simulink model "EnergyDemandBackward"  (R2022b)
settings: Solver=ode4  StartTime=0.0  StopTime=tCycle_s(end)  FixedStep=1  RelTol=1e-3  EnableMultiTasking=on
undefined symbols (not defined in the file or in its folder): areaVeh, distRange_km, etaRec, facCw, facRoll, g, massVeh, rhoAir, tCycle_s, velCycle_kph
libraries: simulink x2
settings Model: Creator=raschul  LastModifiedBy=schuler
settings SolverCC: AlgebraicLoopSolver=TrustRegion
settings DataIOCC: LimitDataPoints=on  SaveFormat=Array  SignalLoggingSaveFormat=ModelDataLogs  ReturnWorkspaceOutputs=off
settings OptimizationCC: ExpressionDepthLimit=2147483647  LifeSpan=inf
settings DebuggingCC: UnderspecifiedInitializationDetection=Classic  MergeDetectMultiDrivingBlocksExec=none  SolverPrmCheckMsg=warning  FcnCallInpInsideContextMsg=warning  UnconnectedInputMsg=warning  UnconnectedOutputMsg=warning  UnconnectedLineMsg=warning  AllowSymbolicDim=off  StateNameClashWarn=warning  SFUnexpectedBacktrackingDiag=warning  SFNoUnconditionalDefaultTransitionDiag=warning  SFExecutionAtInitializationDiag=none  SFMachineParentedDataDiag=warning  ArithmeticOperatorsInVariantConditions=warning
settings HardwareCC: ProdBitPerPointer=32  ProdBitPerSizeT=32  ProdBitPerPtrDiffT=32  ProdLargestAtomicFloat=None  ProdIntDivRoundTo=Undefined  ProdEndianess=Unspecified  ProdWordSize=32  ProdHWDeviceType=32-bit Generic
settings ModelReferenceCC: EnableRefExpFcnMdlSchedulingChecks=on  PropagateSignalLabelsOutOfModel=off
settings SFSimCC: SimUseLocalCustomCode=off  CustomCodeUndefinedFunction=UseInterfaceOnly
settings RTWCC: RTWUseLocalCustomCode=off
settings CodeAppCC: StateflowObjectComments=on
settings GRTTargetCC: TargetLangStandard=C89/C90 (ANSI)  CombineOutputUpdateFcns=off  GRTInterface=on
settings ConfigComp: CovMetricSettings=dw  CovSaveCumulativeToWorkspaceVar=on  CovSaveSingleToWorkspaceVar=on  CovExternalEMLEnable=off

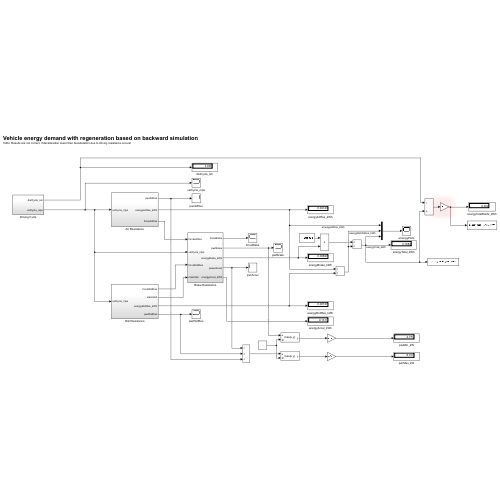
[thumbnail: Simulink's stored preview of the top-level diagram]
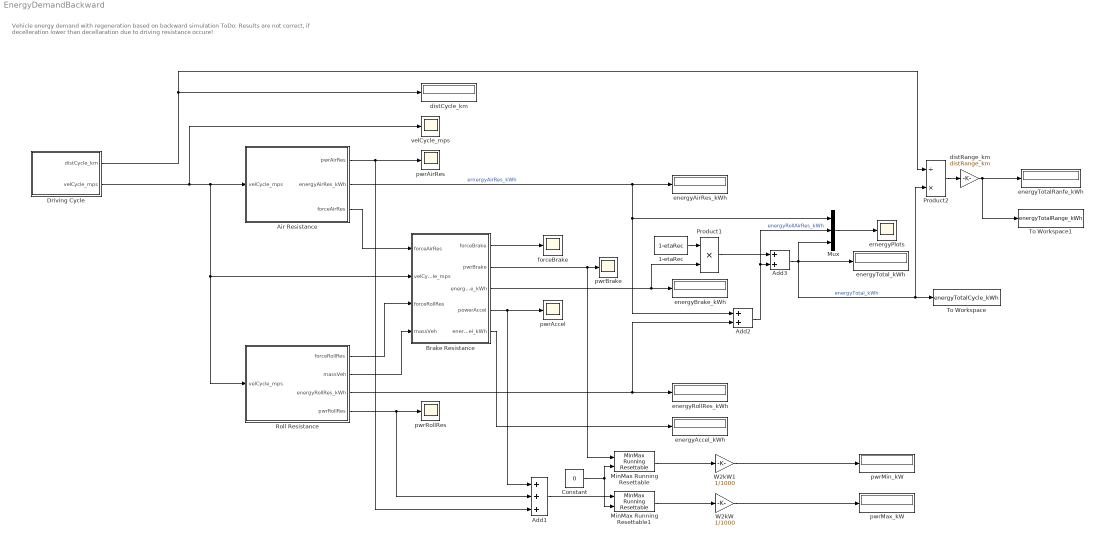
== system EnergyDemandBackward ==
  note: Vehicle energy demand with regeneration based on backward simulation
      | ToDo: Results are not correct, if decelleration lower than decellaration due to driving resistance occure!
  1-etaRec : Constant  Value=1-etaRec
  Add1 : Sum  Inputs=+++
  Add2 : Sum
  Add3 : Sum
  Air Resistance : Subsystem
  Brake Resistance : Subsystem
  Constant : Constant  Value=0
  Driving Cycle : Subsystem
  MinMax Running Resettable : simulink/Math Operations/MinMax Running Resettable  Function=max  vinit=0.0
  MinMax Running Resettable1 : simulink/Math Operations/MinMax Running Resettable  Function=max  vinit=0.0
  Mux : Mux  Inputs=3
  Product1 : Product  RndMeth=Zero
  Product2 : Product  Inputs=/*  RndMeth=Zero
  Roll Resistance : Subsystem
  To Workspace : ToWorkspace  VariableName=energyTotalCycle_kWh  SaveFormat=Timeseries  SampleTime=-1
  To Workspace1 : ToWorkspace  VariableName=energyTotalRange_kWh  SaveFormat=Timeseries  SampleTime=-1
  W2kW : Gain  Gain=1/1000
  W2kW1 : Gain  Gain=1/1000
  distCycle_km : Display
  distRange_km : Gain  Gain=distRange_km
  energyAccel_kWh : Display
  energyAirRes_kWh : Display
  energyBrake_kWh : Display
  energyRollRes_kWh : Display
  energyTotalRanfe_kWh : Display
  energyTotal_kWh : Display
  ernergyPlots : Scope
  forceBrake : Scope
  pwrAccel : Scope
  pwrAirRes : Scope
  pwrBrake : Scope
  pwrMax_kW : Display
  pwrMin_kW : Display
  pwrRollRes : Scope
  velCycle_mps : Scope
  wires:
  Driving Cycle/2(velCycle_mps) -> velCycle_mps/1, Roll Resistance/1(velCycle_mps), Brake Resistance/2(velCycle_mps), Air Resistance/1(velCycle_mps)
  Air Resistance/2(energyAirRes_kWh) -> Mux/1, Add2/1, energyAirRes_kWh/1  "ernergyAirRes_kWh"
  Roll Resistance/3(energyRollRes_kWh) -> Add2/2, energyRollRes_kWh/1
  Add2/1 -> Mux/2, Add3/2  "energyRollAirRes_kWh"
  Add3/1 -> Product2/2, To Workspace/1, Mux/3, energyTotal_kWh/1  "energyTotal_kWh"
  Mux/1 -> ernergyPlots/1
  Air Resistance/1(pwrAirRes) -> Add1/3, pwrAirRes/1
  Air Resistance/3(forceAirRes) -> Brake Resistance/1(forceAirRes)
  Roll Resistance/4(pwrRollRes) -> Add1/2, pwrRollRes/1
  Roll Resistance/1(forceRollRes) -> Brake Resistance/3(forceRollRes)
  Roll Resistance/2(massVeh) -> Brake Resistance/4(massVeh)
  Brake Resistance/1(forceBrake) -> forceBrake/1
  Brake Resistance/2(pwrBrake) -> MinMax Running Resettable/1, pwrBrake/1
  Driving Cycle/1(distCycle_km) -> Product2/1, distCycle_km/1
  Brake Resistance/4(powerAccel) -> pwrAccel/1, Add1/1
  Add1/1 -> MinMax Running Resettable1/1
  MinMax Running Resettable1/1 -> W2kW/1
  W2kW/1 -> pwrMax_kW/1
  MinMax Running Resettable/1 -> W2kW1/1
  W2kW1/1 -> pwrMin_kW/1
  Constant/1 -> MinMax Running Resettable1/2, MinMax Running Resettable/2
  Product1/1 -> Add3/1
  Brake Resistance/5(energyAccel_kWh) -> energyAccel_kWh/1
  1-etaRec/1 -> Product1/1
  Brake Resistance/3(energyBrake_kWh) -> Product1/2, energyBrake_kWh/1
  Product2/1 -> distRange_km/1
  distRange_km/1 -> To Workspace1/1, energyTotalRanfe_kWh/1

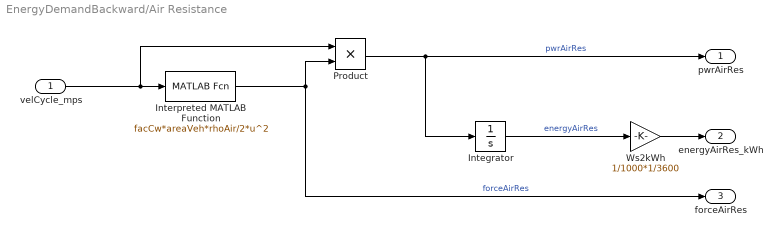
== system EnergyDemandBackward/Air Resistance ==
  velCycle_mps : Inport
  Integrator : Integrator
  Interpreted MATLAB Function : MATLABFcn  MATLABFcn=facCw*areaVeh*rhoAir/2*u^2
  Product : Product  RndMeth=Zero
  Ws2kWh : Gain  Gain=1/1000*1/3600
  pwrAirRes : Outport  VectorParamsAs1DForOutWhenUnconnected=off
  energyAirRes_kWh : Outport  Port=2  VectorParamsAs1DForOutWhenUnconnected=off
  forceAirRes : Outport  Port=3  VectorParamsAs1DForOutWhenUnconnected=off
  wires:
  Interpreted MATLAB Function/1 -> Product/2, forceAirRes/1  "forceAirRes"
  Product/1 -> Integrator/1, pwrAirRes/1  "pwrAirRes"
  Integrator/1 -> Ws2kWh/1  "energyAirRes"
  velCycle_mps/1 -> Product/1, Interpreted MATLAB Function/1
  Ws2kWh/1 -> energyAirRes_kWh/1

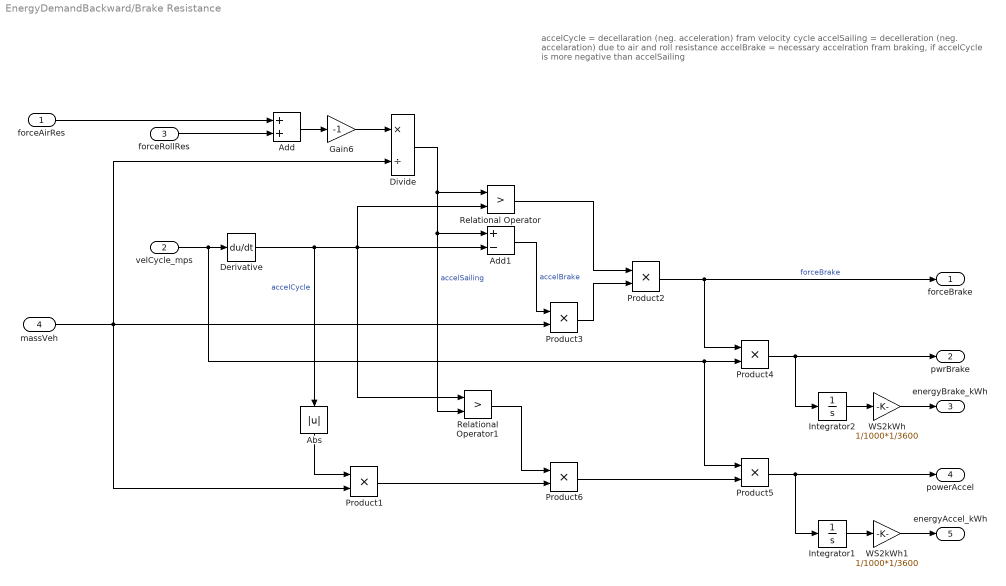
== system EnergyDemandBackward/Brake Resistance ==
  note: accelCycle = decellaration (neg. acceleration) fram velocity cycle
      | accelSailing = decelleration (neg. accelaration) due to air and roll resistance
      | accelBrake = necessary accelration fram braking, if accelCycle is more negative than accelSailing
  forceAirRes : Inport
  velCycle_mps : Inport  Port=2
  forceRollRes : Inport  Port=3
  massVeh : Inport  Port=4
  Abs : Abs  SaturateOnIntegerOverflow=off
  Add : Sum
  Add1 : Sum  Inputs=+-
  Derivative : Derivative
  Divide : Product  Inputs=*/
  Gain6 : Gain  Gain=-1
  Integrator1 : Integrator
  Integrator2 : Integrator
  Product{1..6} (6 alike) : Product  RndMeth=Zero
  Relational Operator : RelationalOperator  Operator=>  OutDataTypeStr=boolean  InputSameDT=off
  Relational Operator1 : RelationalOperator  Operator=>  OutDataTypeStr=boolean  InputSameDT=off
  WS2kWh : Gain  Gain=1/1000*1/3600
  WS2kWh1 : Gain  Gain=1/1000*1/3600
  forceBrake : Outport  VectorParamsAs1DForOutWhenUnconnected=off
  pwrBrake : Outport  Port=2  VectorParamsAs1DForOutWhenUnconnected=off
  energyBrake_kWh : Outport  Port=3  VectorParamsAs1DForOutWhenUnconnected=off
  powerAccel : Outport  Port=4  VectorParamsAs1DForOutWhenUnconnected=off
  energyAccel_kWh : Outport  Port=5  VectorParamsAs1DForOutWhenUnconnected=off
  wires:
  Derivative/1 -> Abs/1, Relational Operator1/1, Relational Operator/2, Add1/2  "accelCycle"
  Add/1 -> Gain6/1
  Gain6/1 -> Divide/1
  Divide/1 -> Relational Operator1/2, Add1/1, Relational Operator/1  "accelSailing"
  Relational Operator/1 -> Product2/1
  Add1/1 -> Product3/1  "accelBrake"
  Product3/1 -> Product2/2
  massVeh/1 -> Product1/2, Product3/2, Divide/2
  velCycle_mps/1 -> Product5/1, Product4/2, Derivative/1
  forceAirRes/1 -> Add/1
  forceRollRes/1 -> Add/2
  Product2/1 -> Product4/1, forceBrake/1  "forceBrake"
  Integrator2/1 -> WS2kWh/1
  Product4/1 -> pwrBrake/1, Integrator2/1
  WS2kWh/1 -> energyBrake_kWh/1
  Relational Operator1/1 -> Product6/1
  Product1/1 -> Product6/2
  Product6/1 -> Product5/2
  Integrator1/1 -> WS2kWh1/1
  Product5/1 -> Integrator1/1, powerAccel/1
  WS2kWh1/1 -> energyAccel_kWh/1
  Abs/1 -> Product1/1

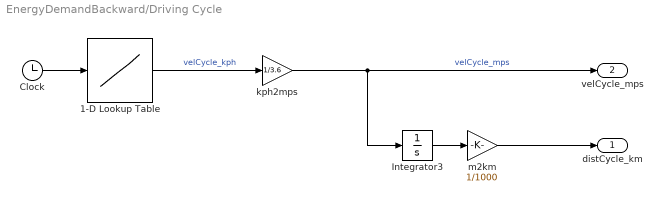
== system EnergyDemandBackward/Driving Cycle ==
  1-D Lookup Table : Lookup_n-D  NumberOfTableDimensions=1  BreakpointsForDimension1=tCycle_s  Table=velCycle_kph  RndMeth=Simplest
  Clock : Clock
  Integrator3 : Integrator
  kph2mps : Gain  Gain=1/3.6
  m2km : Gain  Gain=1/1000
  distCycle_km : Outport  VectorParamsAs1DForOutWhenUnconnected=off
  velCycle_mps : Outport  Port=2  VectorParamsAs1DForOutWhenUnconnected=off
  wires:
  1-D Lookup Table/1 -> kph2mps/1  "velCycle_kph"
  Clock/1 -> 1-D Lookup Table/1
  kph2mps/1 -> Integrator3/1, velCycle_mps/1  "velCycle_mps"
  Integrator3/1 -> m2km/1
  m2km/1 -> distCycle_km/1

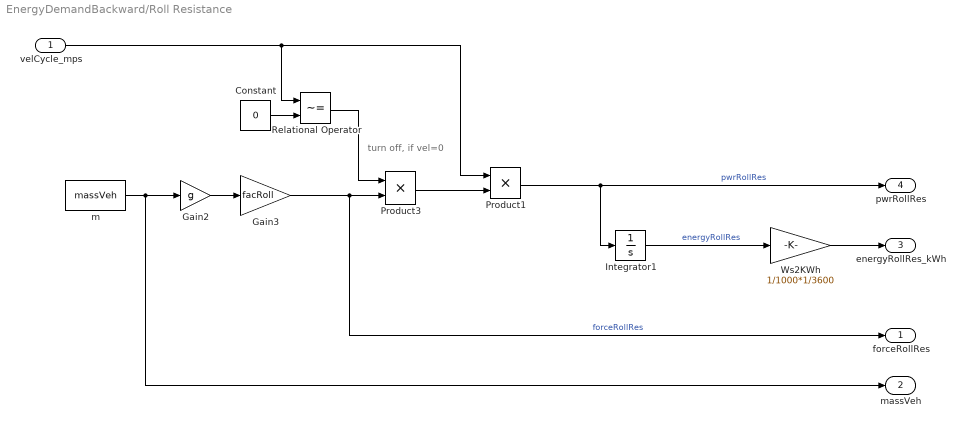
== system EnergyDemandBackward/Roll Resistance ==
  note: turn off, if vel=0
  velCycle_mps : Inport
  Constant : Constant  Value=0
  Gain2 : Gain  Gain=g
  Gain3 : Gain  Gain=facRoll
  Integrator1 : Integrator
  Product1 : Product  RndMeth=Zero
  Product3 : Product  RndMeth=Zero
  Relational Operator : RelationalOperator  Operator=~=  OutDataTypeStr=boolean  InputSameDT=off
  Ws2KWh : Gain  Gain=1/1000*1/3600
  m : Constant  Value=massVeh
  forceRollRes : Outport  VectorParamsAs1DForOutWhenUnconnected=off
  massVeh : Outport  Port=2  VectorParamsAs1DForOutWhenUnconnected=off
  energyRollRes_kWh : Outport  Port=3  VectorParamsAs1DForOutWhenUnconnected=off
  pwrRollRes : Outport  Port=4  VectorParamsAs1DForOutWhenUnconnected=off
  wires:
  m/1 -> Gain2/1, massVeh/1
  Gain2/1 -> Gain3/1
  Product1/1 -> Integrator1/1, pwrRollRes/1  "pwrRollRes"
  Integrator1/1 -> Ws2KWh/1  "energyRollRes"
  Ws2KWh/1 -> energyRollRes_kWh/1
  Relational Operator/1 -> Product3/1
  velCycle_mps/1 -> Product1/1, Relational Operator/1
  Constant/1 -> Relational Operator/2
  Gain3/1 -> forceRollRes/1, Product3/2  "forceRollRes"
  Product3/1 -> Product1/2
